simulink model "Modelle"  (R2021a)
settings: Solver=VariableStepAuto  StartTime=0.0  StopTime=1  FixedStep=0.001  RelTol=1e-10  EnableMultiTasking=on
values from neighbouring files (symbols this model uses):
  g = block.DialogPrm(1).Data    [sFunModell.m]
  l1 = block.DialogPrm(4).Data    [sFunModell.m]
  l2 = block.DialogPrm(5).Data    [sFunModell.m]
  m1 = block.DialogPrm(2).Data    [sFunModell.m]
  m2 = block.DialogPrm(3).Data    [sFunModell.m]
  Rp1 = block.DialogPrm(6).Data    [sFunModell.m]
  Rp2 = block.DialogPrm(7).Data    [sFunModell.m]
settings Model: Creator=gong  LastModifiedBy=aless
settings SolverCC: AlgebraicLoopSolver=TrustRegion
settings DataIOCC: SaveFormat=StructureWithTime  ReturnWorkspaceOutputs=off
settings OptimizationCC: LifeSpan=inf
settings DebuggingCC: SFUnexpectedBacktrackingDiag=warning  SFNoUnconditionalDefaultTransitionDiag=warning  SFExecutionAtInitializationDiag=none  SFMachineParentedDataDiag=warning  ArithmeticOperatorsInVariantConditions=warning
settings HardwareCC: ProdBitPerPointer=32  ProdBitPerSizeT=32  ProdBitPerPtrDiffT=32  ProdLargestAtomicFloat=None  ProdIntDivRoundTo=Undefined  ProdEndianess=Unspecified  ProdWordSize=32  ProdHWDeviceType=32-bit Generic
settings ModelReferenceCC: PropagateSignalLabelsOutOfModel=off
settings SFSimCC: SimUseLocalCustomCode=off  CustomCodeUndefinedFunction=UseInterfaceOnly
settings RTWCC: RTWUseLocalCustomCode=off
settings CodeAppCC: StateflowObjectComments=on
settings GRTTargetCC: TargetLangStandard=C89/C90 (ANSI)
settings ConfigComp: CovMetricSettings=dw  CovSaveCumulativeToWorkspaceVar=on  CovSaveSingleToWorkspaceVar=on  CovExternalEMLEnable=off

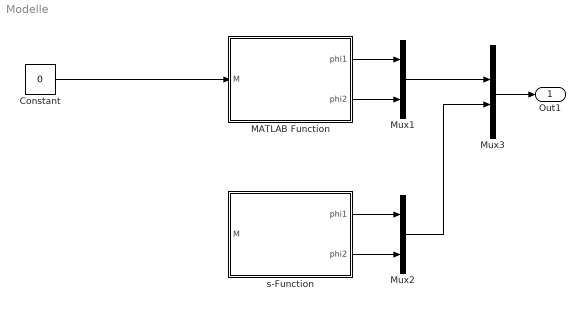
== system Modelle ==
  Constant : Constant  Value=0
  MATLAB Function : Subsystem
  Mux1 : Mux  Inputs=2
  Mux2 : Mux  Inputs=2
  Mux3 : Mux
  s-Function : Subsystem
  Out1 : Outport
  wires:
  MATLAB Function/1(phi1) -> Mux1/1
  MATLAB Function/2(phi2) -> Mux1/2
  s-Function/1(phi1) -> Mux2/1
  s-Function/2(phi2) -> Mux2/2
  Mux1/1 -> Mux3/2
  Mux2/1 -> Mux3/3
  Mux3/1 -> Out1/1
  Constant/1 -> MATLAB Function/1(M)

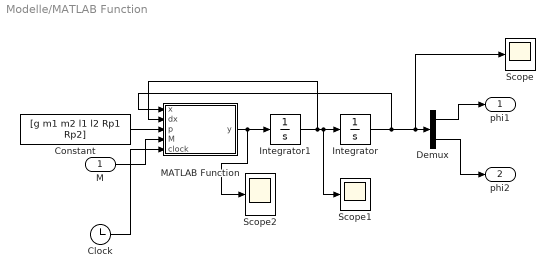
== system Modelle/MATLAB Function ==
  M : Inport
  Clock : Clock
      settings: Decimation=1000
  Constant : Constant  Value=[g m1 m2 l1 l2 Rp1 Rp2]
  Demux : Demux  Outputs=2
  Integrator : Integrator
  Integrator1 : Integrator
  MATLAB Function : MATLAB Function  TreatAsAtomicUnit=on
  Scope : Scope
  Scope1 : Scope
  Scope2 : Scope
  phi1 : Outport
  phi2 : Outport  Port=2
  wires:
  Constant/1 -> MATLAB Function/3(p)
  M/1 -> MATLAB Function/4(M)
  Demux/1 -> phi1/1
  Demux/2 -> phi2/1
  MATLAB Function/1(y) -> Scope2/1, Integrator1/1
  Integrator1/1 -> MATLAB Function/2(dx), Scope1/1, Integrator/1
  Integrator/1 -> MATLAB Function/1(x), Scope/1, Demux/1
  Clock/1 -> MATLAB Function/5(clock)

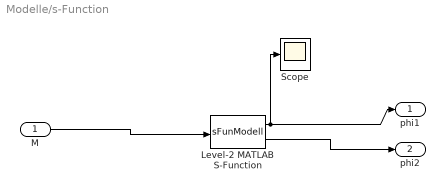
== system Modelle/s-Function ==
  M : Inport
  Level-2 MATLAB S-Function : M-S-Function  FunctionName=sFunModell  Parameters=g, m1, m2, l1, l2, Rp1, Rp2
  Scope : Scope
  phi1 : Outport
  phi2 : Outport  Port=2
  wires:
  M/1 -> Level-2 MATLAB S-Function/1
  Level-2 MATLAB S-Function/1 -> Scope/1, phi1/1
  Level-2 MATLAB S-Function/2 -> phi2/1

== matlab function Modelle/MATLAB Function/MATLAB Function ==
  data: x input; y output size=[1 2]; dx input; p input; M input; clock input
function y = fcn(x,dx, p, M, clock)
g=p(1);
m1=p(2);
m2=p(3);
l1=p(4);
l2=p(5);
Rp1=p(6);
Rp2=p(7);

    
phi1=x(1);
phi2=x(2);
dphi1=dx(1);
dphi2=dx(2);


ddphi1= -(24*(26*Rp1*dphi1*l2 - 26*M*l2 + 26*Rp2*dphi1*l2 - 26*Rp2*dphi2*l2 + 48*Rp2*dphi1*l1*cos(phi1 - phi2)...
    - 48*Rp2*dphi2*l1*cos(phi1 - phi2) + 12*g*l1*l2*m2*sin(phi1 - 2*phi2)...
    + 12*dphi1^2*l1^2*l2*m2*sin(2*phi1 - 2*phi2) + 13*dphi2^2*l1*l2^2*m2*sin(phi1 - phi2)...
    + 27*g*l1*l2*m2*sin(phi1)))/(l1^2*l2*(169*m1 + 336*m2 - 288*m2*cos(2*phi1 - 2*phi2)))


ddphi2=(24*(26*Rp2*dphi1*l1*m1 - 48*M*l2*m2*cos(phi1 - phi2) + 96*Rp2*dphi1*l1*m2...
    - 26*Rp2*dphi2*l1*m1 - 96*Rp2*dphi2*l1*m2 + 48*dphi1^2*l1^2*l2*m2^2*sin(phi1 - phi2)...
    - 12*g*l1*l2*m2^2*sin(phi2) + 12*dphi2^2*l1*l2^2*m2^2*sin(2*phi1 - 2*phi2)...
    + 36*g*l1*l2*m2^2*sin(2*phi1 - phi2) + 48*Rp1*dphi1*l2*m2*cos(phi1 - phi2)...
    + 48*Rp2*dphi1*l2*m2*cos(phi1 - phi2) - 48*Rp2*dphi2*l2*m2*cos(phi1 - phi2)...
    + 13*dphi1^2*l1^2*l2*m1*m2*sin(phi1 - phi2) - 13*g*l1*l2*m1*m2*sin(phi2)))...
    /(l1*l2^2*m2*(169*m1 + 336*m2 - 288*m2*cos(2*phi1 - 2*phi2)))





y = [ddphi1, ddphi2];
